simulink model "sim_chua_lin_ctrl_2014"  (R2014a)
settings: Solver=ode23t  SolverMode=SingleTasking  StartTime=0.0  StopTime=tfin  RelTol=1e-3
values from neighbouring files (symbols this model uses):
  C = [0 1 0]    [main_chua_lin_ctrl.m]
  K = place(A,g,[-1,-2,-3])    [main_chua_lin_ctrl.m]
  KI = place(Aa,Ba,-(1:4))    [main_chua_lin_ctrl.m]
  x0 = randn(3,1)*0    [main_chua_lin_ctrl.m]
undefined symbols (not defined in the file or in its folder): fg_chua
libraries: cstblocks x1
settings Model: CovMetricSettings=dwe  CovHtmlReporting=off  covSaveCumulativeToWorkspaceVar=off  CovSaveSingleToWorkspaceVar=off  CovExternalEMLEnable=on  CovSFcnEnable=on  Creator=carlonovara  LastModifiedBy=carlonovara
settings DataIOCC: LimitDataPoints=off  SaveFormat=StructureWithTime
settings DebuggingCC: MergeDetectMultiDrivingBlocksExec=error  SolverPrmCheckMsg=none  FrameProcessingCompatibilityMsg=error  SFUnexpectedBacktrackingDiag=error  SFNoUnconditionalDefaultTransitionDiag=error
settings HardwareCC: ProdBitPerPointer=64  ProdLargestAtomicFloat=Float  ProdIntDivRoundTo=Zero  ProdEndianess=LittleEndian  ProdHWDeviceType=Specified
settings ModelReferenceCC: PropagateSignalLabelsOutOfModel=on
settings GRTTargetCC: TargetLangStandard=C99 (ISO)  GeneratePreprocessorConditionals=Use local settings

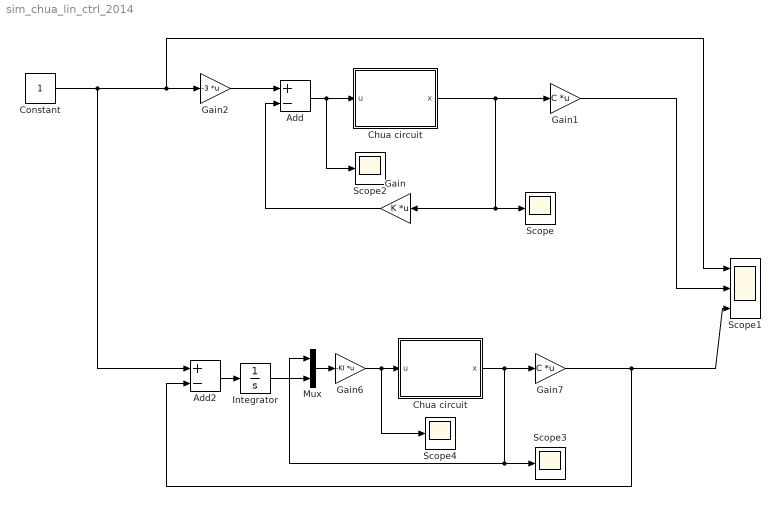
== system sim_chua_lin_ctrl_2014 ==
  Add : Sum  Inputs=+-
  Add2 : Sum  Inputs=+-
  Chua circuit : Subsystem
  "Chua circuit " : Subsystem
  Constant : Constant
  Gain : Gain  Gain=K  Multiplication=Matrix(K*u)
  Gain1 : Gain  Gain=C  Multiplication=Matrix(K*u)
  Gain2 : Gain  Gain=-3  Multiplication=Matrix(K*u)
  Gain6 : Gain  Gain=-KI  Multiplication=Matrix(K*u)
  Gain7 : Gain  Gain=C  Multiplication=Matrix(K*u)
  Integrator : Integrator
  Mux : Mux  Inputs=2
  Scope{,2..4} (4 alike) : Scope
      Scope settings: TimeRange=auto  MaxDataPoints=5000  SaveToWorkspace=off  SaveName=ScopeData  YMin=-15.11616  YMax=3.43537  SampleTime=-1
      Scope2 settings: TimeRange=auto  MaxDataPoints=5000  SaveToWorkspace=off  YMin=-1.14081  YMax=5.19414  SampleTime=-1
      Scope3 settings: TimeRange=auto  MaxDataPoints=5000  SaveToWorkspace=off  YMin=-185.39095  YMax=24.3185  SampleTime=-1
      Scope4 settings: TimeRange=auto  MaxDataPoints=5000  SaveToWorkspace=off  SaveName=ScopeData2  YMin=-21.5926  YMax=182.48172  SampleTime=-1
  Scope1 : Scope  NumInputPorts=3
      settings: TimeRange=auto  MaxDataPoints=5000  SaveToWorkspace=off  YMin=-0.41876~-5~-5  YMax=1.15764~5~5  SampleTime=-1
  wires:
  Chua circuit/1(x) -> Gain/1, Scope/1, Gain1/1
  Add/1 -> Scope2/1, Chua circuit/1(u)
  Gain/1 -> Add/2
  Gain2/1 -> Add/1
  Gain1/1 -> Scope1/2
  Gain6/1 -> Scope4/1, "Chua circuit "/1(u)
  Mux/1 -> Gain6/1
  "Chua circuit "/1(x) -> Mux/1, Scope3/1, Gain7/1
  Add2/1 -> Integrator/1
  Gain7/1 -> Scope1/3, Add2/2
  Integrator/1 -> Mux/2
  Constant/1 -> Add2/1, Scope1/1, Gain2/1

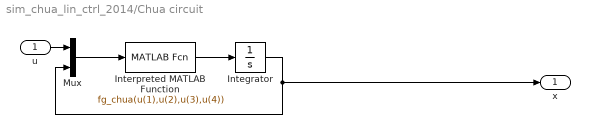
== system sim_chua_lin_ctrl_2014/Chua circuit ==
  u : Inport
  Integrator : Integrator  InitialCondition=x0
  Interpreted MATLAB Function : MATLABFcn  MATLABFcn=fg_chua(u(1),u(2),u(3),u(4))  OutputDimensions=3
  Mux : Mux  Inputs=2
  x : Outport
  wires:
  u/1 -> Mux/1
  Interpreted MATLAB Function/1 -> Integrator/1
  Integrator/1 -> x/1, Mux/2
  Mux/1 -> Interpreted MATLAB Function/1

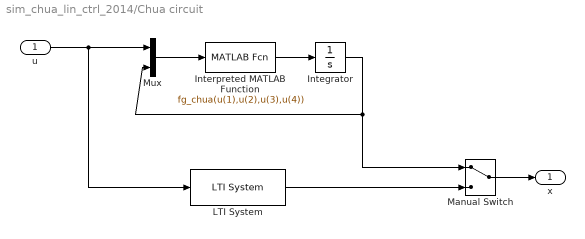
== system sim_chua_lin_ctrl_2014/Chua circuit  ==
  u : Inport
  Integrator : Integrator  InitialCondition=x0
  Interpreted MATLAB Function : MATLABFcn  MATLABFcn=fg_chua(u(1),u(2),u(3),u(4))  OutputDimensions=3
  LTI System : cstblocks/LTI System  sys=M  IC=[]
  Manual Switch : ManualSwitch
  Mux : Mux  Inputs=2
  x : Outport
  wires:
  Mux/1 -> Interpreted MATLAB Function/1
  Integrator/1 -> Mux/2, Manual Switch/1
  Interpreted MATLAB Function/1 -> Integrator/1
  u/1 -> LTI System/1, Mux/1
  Manual Switch/1 -> x/1
  LTI System/1 -> Manual Switch/2
